simulink model "anglehigh_stab"  (R2017b)
settings: Solver=ode45  StartTime=0.0  StopTime=time_end  RelTol=1e-3  EnableMultiTasking=on
values from neighbouring files (symbols this model uses):
  alpha_initial = 0    [run.m]
  g = 9.8    [run.m]
  gamma = (k)/(2*m*r)    (= 6.57462195924)    [run.m]
  k = 0.8    [run.m]
  m = 0.078    [run.m]
  W_initial = 0    [run.m]
  x_initial = 0.5    [run.m]
  z0 = 3    [run.m]
  z_initial = 0.5    [run.m]
undefined symbols (not defined in the file or in its folder): magnitude
settings Model: Creator=Subject 1482  LastModifiedBy=Subject 1482
settings DataIOCC: LimitDataPoints=on  SaveFormat=Array
settings OptimizationCC: LifeSpan=inf
settings DebuggingCC: SFUnexpectedBacktrackingDiag=warning  SFNoUnconditionalDefaultTransitionDiag=warning  SFExecutionAtInitializationDiag=none
settings HardwareCC: ProdBitPerPointer=32  ProdBitPerSizeT=32  ProdBitPerPtrDiffT=32  ProdLargestAtomicFloat=None  ProdIntDivRoundTo=Undefined  ProdEndianess=Unspecified  ProdWordSize=32  ProdHWDeviceType=32-bit Generic
settings ModelReferenceCC: PropagateSignalLabelsOutOfModel=off
settings CodeAppCC: StateflowObjectComments=on
settings GRTTargetCC: TargetLangStandard=C89/C90 (ANSI)  GeneratePreprocessorConditionals=Disable all
settings ConfigComp: CovMetricSettings=dw  CovHtmlReporting=on  CovSaveCumulativeToWorkspaceVar=on  CovSaveSingleToWorkspaceVar=on  CovExternalEMLEnable=off

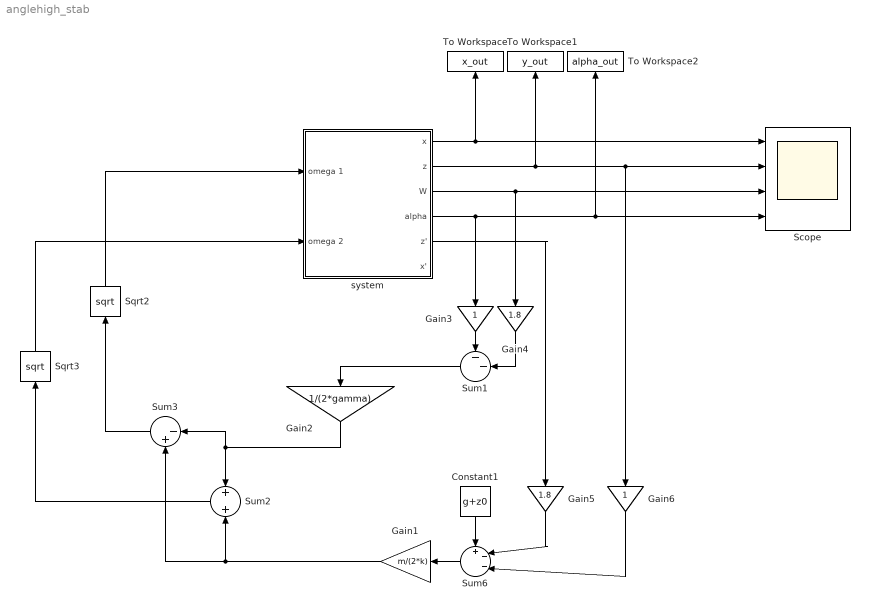
== system anglehigh_stab ==
  Constant1 : Constant  Value=g+z0
  Gain1 : Gain  Gain=m/(2*k)
  Gain2 : Gain  Gain=1/(2*gamma)
  Gain3 : Gain
  Gain4 : Gain  Gain=1.8
  Gain5 : Gain  Gain=1.8
  Gain6 : Gain
  Scope : Scope  NumInputPorts=4
  Sqrt2 : Sqrt  SaturateOnIntegerOverflow=on
  Sqrt3 : Sqrt  SaturateOnIntegerOverflow=on
  Sum1 : Sum  Inputs=--|
  Sum2 : Sum
  Sum3 : Sum  Inputs=|-+
  Sum6 : Sum  Inputs=+--|
  To Workspace : ToWorkspace  VariableName=x_out  SaveFormat=Timeseries  SampleTime=-1
  To Workspace1 : ToWorkspace  VariableName=y_out  SaveFormat=Timeseries  SampleTime=-1
  To Workspace2 : ToWorkspace  VariableName=alpha_out  SaveFormat=Timeseries  SampleTime=-1
  system : Subsystem
  wires:
  system/1(x) -> To Workspace/1, Scope/1
  system/2(z) -> To Workspace1/1, Gain6/1, Scope/2
  system/3(W) -> Gain4/1, Scope/3
  system/4(alpha) -> Scope/4, To Workspace2/1, Gain3/1
  Sqrt2/1 -> system/1(omega 1)
  Sqrt3/1 -> system/2(omega 2)
  Constant1/1 -> Sum6/1
  Sum6/1 -> Gain1/1
  system/5(z') -> Gain5/1
  Sum1/1 -> Gain2/1
  Gain2/1 -> Sum3/1, Sum2/1
  Sum2/1 -> Sqrt3/1
  Sum3/1 -> Sqrt2/1
  Gain3/1 -> Sum1/1
  Gain4/1 -> Sum1/2
  Gain5/1 -> Sum6/2
  Gain6/1 -> Sum6/3
  Gain1/1 -> Sum2/2, Sum3/2

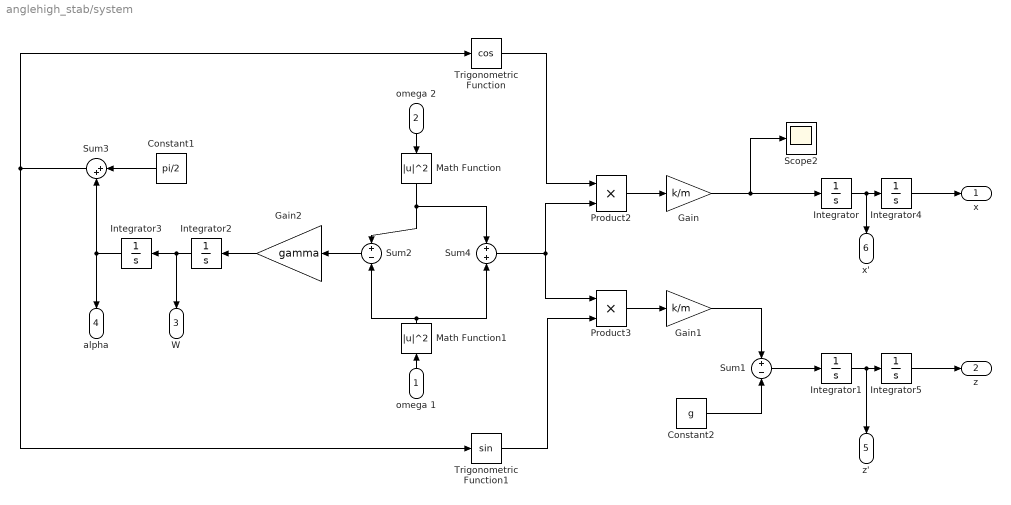
== system anglehigh_stab/system ==
  omega 1 : Inport
  omega 2 : Inport  Port=2
  Constant1 : Constant  Value=pi/2
  Constant2 : Constant  Value=g
  Gain : Gain  Gain=k/m
  Gain1 : Gain  Gain=k/m
  Gain2 : Gain  Gain=gamma
  Integrator : Integrator
  Integrator1 : Integrator
  Integrator2 : Integrator  InitialCondition=W_initial
  Integrator3 : Integrator  InitialCondition=alpha_initial
  Integrator4 : Integrator  InitialCondition=x_initial
  Integrator5 : Integrator  InitialCondition=z_initial
  Math Function : Math  Operator=magnitude^2  SaturateOnIntegerOverflow=on
  Math Function1 : Math  Operator=magnitude^2  SaturateOnIntegerOverflow=on
  Product2 : Product
  Product3 : Product
  Scope2 : Scope
  Sum1 : Sum  Inputs=+-
  Sum2 : Sum  Inputs=+-
  Sum3 : Sum  Inputs=|++
  Sum4 : Sum
  Trigonometric Function : Trigonometry  Operator=cos
  Trigonometric Function1 : Trigonometry
  x : Outport
  z : Outport  Port=2
  W : Outport  Port=3
  alpha : Outport  Port=4
  z' : Outport  Port=5
  x' : Outport  Port=6
  wires:
  Constant2/1 -> Sum1/2
  Gain1/1 -> Sum1/1
  Sum1/1 -> Integrator1/1
  Product3/1 -> Gain1/1
  Trigonometric Function/1 -> Product2/1
  Gain2/1 -> Integrator2/1
  Integrator3/1 -> Sum3/2, alpha/1
  Trigonometric Function1/1 -> Product3/2
  Product2/1 -> Gain/1
  Gain/1 -> Scope2/1, Integrator/1
  Integrator2/1 -> W/1, Integrator3/1
  Constant1/1 -> Sum3/1
  Sum3/1 -> Trigonometric Function1/1, Trigonometric Function/1
  Integrator1/1 -> z'/1, Integrator5/1
  Integrator5/1 -> z/1
  Integrator/1 -> x'/1, Integrator4/1
  Integrator4/1 -> x/1
  omega 2/1 -> Math Function/1
  omega 1/1 -> Math Function1/1
  Sum2/1 -> Gain2/1
  Sum4/1 -> Product3/1, Product2/2
  Math Function1/1 -> Sum2/2, Sum4/2
  Math Function/1 -> Sum4/1, Sum2/1
